simulink model "testes_simulink"  (R2022a)
settings: Solver=ode3  StartTime=0.0  StopTime=10.0  FixedStep=1e-3  RelTol=1e-3
libraries: simulink x1
settings Model: Creator=souza  LastModifiedBy=souza

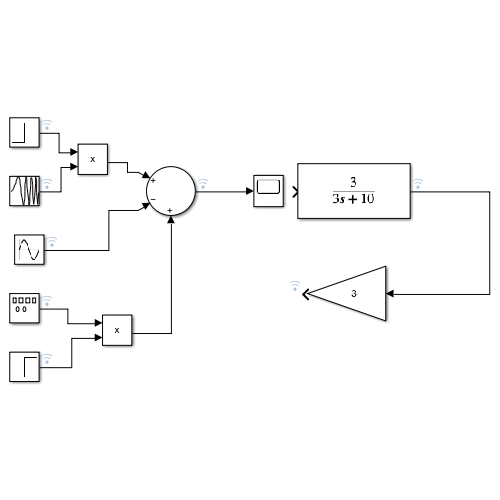
[thumbnail: Simulink's stored preview of the top-level diagram]
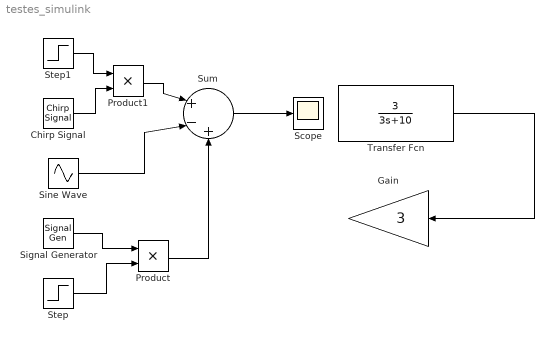
== system testes_simulink ==
  Chirp Signal : simulink/Sources/Chirp Signal  f1=1  T=50  f2=1
  Gain : Gain  Gain=3
  Product : Product
  Product1 : Product
  Scope : Scope
  Signal Generator : SignalGenerator  WaveForm=square  Frequency=6  Units=rad/sec
  Sine Wave : Sin  Amplitude=2  Bias=20  Phase=50  SampleTime=0
  Step : Step  Time=3  After=2  SampleTime=0
  Step1 : Step  Time=8  After=2  SampleTime=0
  Sum : Sum  Inputs=|+-+
  Transfer Fcn : TransferFcn  Numerator=3  Denominator=[3 10]
  wires:
  Transfer Fcn/1 -> Gain/1
  Sum/1 -> Scope/1
  Sine Wave/1 -> Sum/2
  Product/1 -> Sum/3
  Step/1 -> Product/2
  Signal Generator/1 -> Product/1
  Product1/1 -> Sum/1
  Chirp Signal/1 -> Product1/2
  Step1/1 -> Product1/1
